simulink model "EquationOfAStrightLine"  (R2020b)
settings: Solver=VariableStepAuto  StartTime=0.0  StopTime=10.0  RelTol=1e-3
settings Model: Creator=99003759  LastModifiedBy=99003759

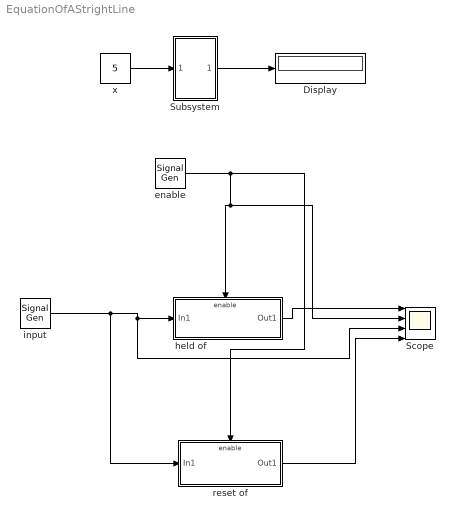
== system EquationOfAStrightLine ==
  Display : Display
  Scope : Scope  NumInputPorts=4
  Subsystem : Subsystem  TreatAsAtomicUnit=on  mask(claculating the value){m=5, c=7}
      mask prompts: m "slop of a line"; c "constant"
      mask help: it used to calculate straight line equation
      mask Help: ltt.com
      mask Display: image('C:\99003759\straight-line.jpg')
  enable : SignalGenerator  WaveForm=square  Frequency=2
  held of : Subsystem
  input : SignalGenerator  Units=rad/sec
  reset of : Subsystem
  x : Constant  Value=5
  wires:
  Subsystem/1(Out1) -> Display/1
  x/1 -> Subsystem/1(In1)
  input/1 -> reset of/1(In1), Scope/3, held of/1(In1)
  held of/1(Out1) -> Scope/1
  reset of/1(Out1) -> Scope/4
  enable/1 -> reset of/Enable, Scope/2, held of/Enable

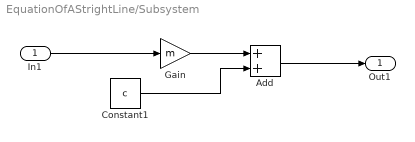
== system EquationOfAStrightLine/Subsystem ==
  In1 : Inport
  Add : Sum
  Constant1 : Constant  Value=c
  Gain : Gain  Gain=m
  Out1 : Outport
  wires:
  Gain/1 -> Add/1
  Constant1/1 -> Add/2
  In1/1 -> Gain/1
  Add/1 -> Out1/1

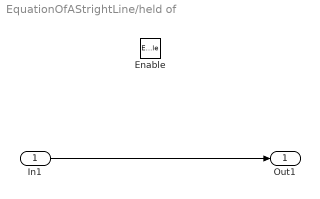
== system EquationOfAStrightLine/held of ==
  In1 : Inport
  Enable : EnablePort
  Out1 : Outport
  wires:
  In1/1 -> Out1/1

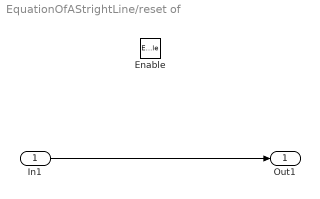
== system EquationOfAStrightLine/reset of ==
  In1 : Inport
  Enable : EnablePort  StatesWhenEnabling=reset
  Out1 : Outport
  wires:
  In1/1 -> Out1/1
